simulink model "PX30"  (R2015b)
settings: Solver=FixedStepAuto  StartTime=0.0  StopTime=3  FixedStep=1  RelTol=1e-3
settings Model: Creator=xmax1946  LastModifiedBy=xmax1946

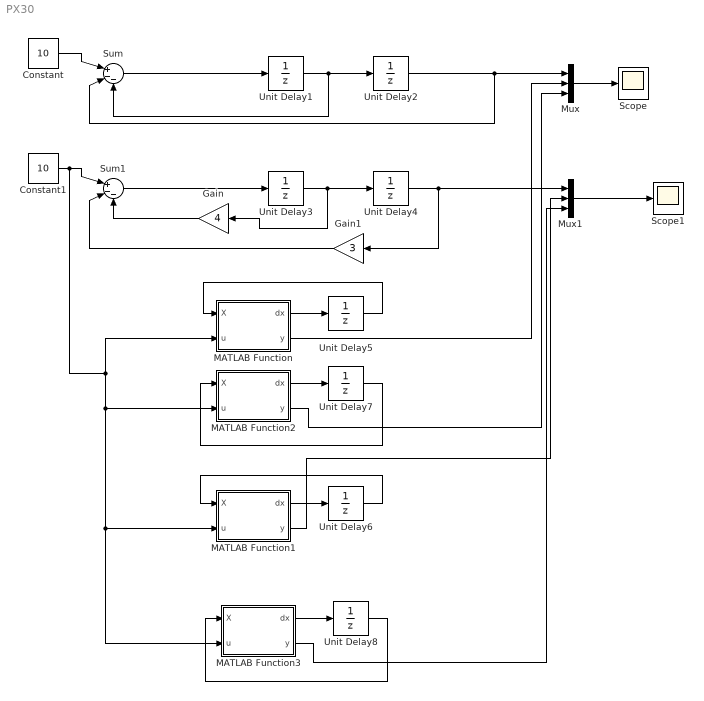
== system PX30 ==
  Constant : Constant  Value=10
  Constant1 : Constant  Value=10
  Gain : Gain  Gain=4
  Gain1 : Gain  Gain=3
  MATLAB Function : MATLAB Function  TreatAsAtomicUnit=on
  MATLAB Function1 : MATLAB Function  TreatAsAtomicUnit=on
  MATLAB Function2 : MATLAB Function  TreatAsAtomicUnit=on
  MATLAB Function3 : MATLAB Function  TreatAsAtomicUnit=on
  Mux : Mux  Inputs=3
  Mux1 : Mux  Inputs=3
  Scope : Scope
  Scope1 : Scope
  Sum : Sum  Inputs=|+--
  Sum1 : Sum  Inputs=|+--
  Unit Delay1 : UnitDelay  InitialCondition=-1  SampleTime=-1
  Unit Delay2 : UnitDelay  InitialCondition=1  SampleTime=-1
  Unit Delay3 : UnitDelay  InitialCondition=-1  SampleTime=-1
  Unit Delay4 : UnitDelay  InitialCondition=2  SampleTime=-1
  Unit Delay5 : UnitDelay  InitialCondition=[10;1]  SampleTime=-1
  Unit Delay6 : UnitDelay  InitialCondition=[1;2]  SampleTime=-1
  Unit Delay7 : UnitDelay  InitialCondition=[-10;1]  SampleTime=-1
  Unit Delay8 : UnitDelay  InitialCondition=[-3;2]  SampleTime=-1
  wires:
  Mux/1 -> Scope/1
  Unit Delay1/1 -> Sum/3, Unit Delay2/1
  Unit Delay2/1 -> Sum/2, Mux/1
  Constant/1 -> Sum/1
  Sum/1 -> Unit Delay1/1
  Mux1/1 -> Scope1/1
  Unit Delay3/1 -> Gain/1, Unit Delay4/1
  Unit Delay4/1 -> Gain1/1, Mux1/1
  Constant1/1 -> MATLAB Function2/2(u), MATLAB Function3/2(u), MATLAB Function1/2(u), MATLAB Function/2(u), Sum1/1
  Sum1/1 -> Unit Delay3/1
  Gain/1 -> Sum1/3
  Gain1/1 -> Sum1/2
  MATLAB Function/1(dx) -> Unit Delay5/1
  MATLAB Function1/1(dx) -> Unit Delay6/1
  Unit Delay5/1 -> MATLAB Function/1(X)
  Unit Delay6/1 -> MATLAB Function1/1(X)
  MATLAB Function/2(y) -> Mux/2
  MATLAB Function1/2(y) -> Mux1/2
  MATLAB Function2/1(dx) -> Unit Delay7/1
  Unit Delay7/1 -> MATLAB Function2/1(X)
  MATLAB Function2/2(y) -> Mux/3
  MATLAB Function3/1(dx) -> Unit Delay8/1
  Unit Delay8/1 -> MATLAB Function3/1(X)
  MATLAB Function3/2(y) -> Mux1/3

== matlab function PX30/MATLAB Function1 ==
  data: X input; dx output; u input; y output
function [dx,y] = fcn(X,u)
A=[0,1;-3,-4];
B=[0;1];
C=[0,1];

dx=A*X+B*u;
y=C*X;

== matlab function PX30/MATLAB Function ==
  data: X input; dx output; u input; y output
function [dx,y]= fcn(X,u)

A=[0,1;-1,-1];
B=[0;1];
C=[0,1];

dx=A*X+B*u;
y=C*X;

== matlab function PX30/MATLAB Function2 ==
  data: X input; dx output; u input; y output
function [dx,y]= fcn(X,u)

A=[0,-1;1,-1];
B=[0;1];
C=[0,1];

dx=A*X+B*u;
y=C*X;

== matlab function PX30/MATLAB Function3 ==
  data: X input; dx output; u input; y output
function [dx,y] = fcn(X,u)
A=[0,-3;1,-4];
B=[0;1];
C=[0,1];

dx=A*X+B*u;
y=C*X;
